simulink subsystem "Controllers"  (R2024b)
settings: Solver=VariableStepAuto  StartTime=0.0  StopTime=10.0  RelTol=1e-3
undefined symbols (not defined in the file): CarrierFreq, dend, DiscIntNeverNeededParam, freq_left, freq_right, Ll, nb_cell, numberOfCell, numd, P_AC, Rl, Tctrl, Ts, V_AC_sec
libraries: powerlib_extras x12, simulink x12
(part 2 of 4)

== system Controllers/pulsegen_VBC1/pulse_gen ==
  Vcell_ref : Inport
  pgmode : Inport  Port=2
  Carrier_generatorgood : Subsystem  Commented=on  mask{fs=freq_right, nr=12*0+10, nb_mod=numberOfCell, x=0, Ts=Ts}
      mask prompts: fs "PWM freqency"; nr "carrier frequence/PWM freq"; nb_mod "nb cell"; x "x_shift (0:nb_cell, better nb_cell/x_shift not integal)"; Ts "time"
      mask init:
      | fc=fs*nr;
      | fx=fc/(1+x/nb_mod/nr);
  Mux4 : Mux  Inputs=6
  PWM : Subsystem
  Unit Delay : UnitDelay  SampleTime=Ts  HasFrameUpgradeWarning=on
  carrier_gen : Subsystem  mask(carrier generation){fc=CarrierFreq, range=[ 1 -1], Ms=numberOfCell, Ns=numberOfCell}
      mask prompts: fc "carrier frequency (Hz)"; range "carrier signal range"; Ms "M signals"; Ns "Enter N if two consecutive signals shifted (1/N) cycle. Enter 1 if all signals are identical."
      mask help:
      | Generating M number of triangle carrier signal(s) at specific frequency.
      | Two consecutive signals are shifted (1/N) cycles.
      |
      | Example 1:
      | put carrier frequency = 1e3, M=1, it outputs 1 triangle carrier signal with frequency of 1k Hz.
      |
      | Example 2:
      | M=3, N=3, output 3 evenly interleaved carrier signals. ( 2nd signal lags  1st signal by 1/3 cycle ).
      |
      | Example 3:
      | M=3, N=-2.5, output 3 carrier signals. (2nd signal advances 1st signal by 1/2.5 cycle).
      |
      | Example 4:
      | M=3, N=1, output 3 identical carrier signals.
      mask init:
      | fc=max(eps,fc); %avoid devided by 0;
      | % Ns=max(eps,Ns); %avoid devided by 0;
      | if Ns==0    %if Ns==0, not interleaved
      |     Ns=1;
      | end;
      | Ms=max(1,floor(Ms))-1;
      | rep_seq_t=[0 0.5 1]/fc;
      | rep_seq_y=[range(1) range(2) range(1)];
      | 
      | 
      | X = [];
      | Y = [];
      | if (length(rep_seq_t) ~= length(rep_seq_y)),
      |   error('Length of time vector and output vector must be the same.')
      | end
      | dbl_rep_seq_t = double(rep_seq_t);
      | dbl_rep_seq_y = double(rep_seq_y);
      | period = max(dbl_rep_seq_t) - min(dbl_rep_seq_t);
      | period = slResolve(sprintf('%0.5g',period), gcbh);
      | [X, Y] = genRepeatingSequenceBlockIconData(dbl_rep_seq_t, dbl_rep_seq_y);
      | Noffset=-[0:Ms]/Ns*period;
      mask Help: web('https://wiki.opal-rt.com/display/MMCDOC/Carrier+Signal+Generation+Block')
      mask Display: plot(X, Y )
  A_pulse : Outport  VectorParamsAs1DForOutWhenUnconnected=off
  NLC : Outport  Port=2  VectorParamsAs1DForOutWhenUnconnected=off
  wires:
  Unit Delay/1 -> A_pulse/1
  carrier_gen/1(Out1) -> Mux4/1, Mux4/2, Mux4/3, Mux4/4, Mux4/5, Mux4/6
  Vcell_ref/1 -> PWM/2(Vcell_ref)
  PWM/1(Upper_gate) -> Unit Delay/1
  Mux4/1 -> PWM/1(carrier)
  pgmode/1 -> PWM/3(pgmode)
  PWM/2(NLCref) -> NLC/1

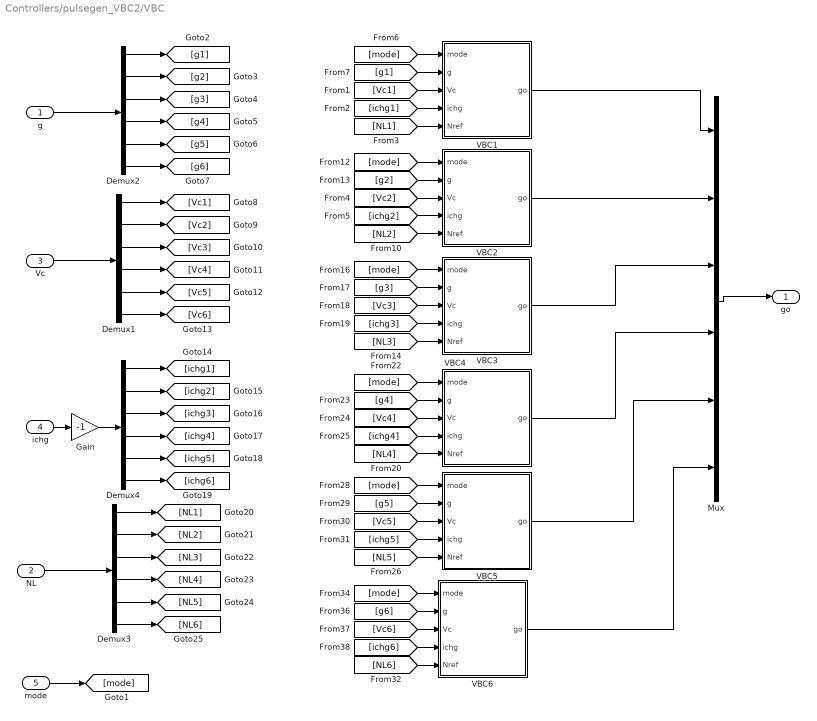
== system Controllers/pulsegen_VBC2/VBC ==
  g : Inport
  NL : Inport  Port=2
  Vc : Inport  Port=3
  ichg : Inport  Port=4
  mode : Inport  Port=5
  Demux{1..4} (4 alike) : Demux  Outputs=6
  Gain : Gain  Gain=-1
  Mux : Mux  Inputs=ones(6,1)*numberOfCell
  VBC1 : Subsystem
  VBC2 : Subsystem
  VBC3 : Subsystem
  VBC4 : Subsystem
  VBC5 : Subsystem
  VBC6 : Subsystem
  go : Outport  VectorParamsAs1DForOutWhenUnconnected=off
  wires:
  [NL6] -> VBC6/5(Nref)
  [ichg6] -> VBC6/4(ichg)
  [Vc6] -> VBC6/3(Vc)
  [g6] -> VBC6/2(g)
  [mode] -> VBC6/1(mode)
  [NL5] -> VBC5/5(Nref)
  [ichg5] -> VBC5/4(ichg)
  [Vc5] -> VBC5/3(Vc)
  [g5] -> VBC5/2(g)
  [mode] -> VBC5/1(mode)
  [NL4] -> VBC4/5(Nref)
  [ichg4] -> VBC4/4(ichg)
  [Vc4] -> VBC4/3(Vc)
  [g4] -> VBC4/2(g)
  [mode] -> VBC4/1(mode)
  [NL3] -> VBC3/5(Nref)
  [ichg3] -> VBC3/4(ichg)
  [Vc3] -> VBC3/3(Vc)
  [g3] -> VBC3/2(g)
  [mode] -> VBC3/1(mode)
  [NL2] -> VBC2/5(Nref)
  [ichg2] -> VBC2/4(ichg)
  [Vc2] -> VBC2/3(Vc)
  [g2] -> VBC2/2(g)
  [mode] -> VBC2/1(mode)
  [NL1] -> VBC1/5(Nref)
  [ichg1] -> VBC1/4(ichg)
  [Vc1] -> VBC1/3(Vc)
  Demux3/6 -> [NL6]
  Demux3/5 -> [NL5]
  Demux3/4 -> [NL4]
  Demux3/3 -> [NL3]
  Demux3/2 -> [NL2]
  Demux3/1 -> [NL1]
  NL/1 -> Demux3/1
  Demux4/6 -> [ichg6]
  Demux4/5 -> [ichg5]
  Demux4/4 -> [ichg4]
  Demux4/3 -> [ichg3]
  Demux4/2 -> [ichg2]
  Demux4/1 -> [ichg1]
  Demux1/6 -> [Vc6]
  Demux1/5 -> [Vc5]
  Demux1/4 -> [Vc4]
  Demux1/3 -> [Vc3]
  Demux1/2 -> [Vc2]
  Demux1/1 -> [Vc1]
  [g1] -> VBC1/2(g)
  Demux2/6 -> [g6]
  Demux2/5 -> [g5]
  Demux2/4 -> [g4]
  Demux2/3 -> [g3]
  Demux2/2 -> [g2]
  Demux2/1 -> [g1]
  [mode] -> VBC1/1(mode)
  mode/1 -> [mode]
  Gain/1 -> Demux4/1
  VBC1/1(go) -> Mux/1
  g/1 -> Demux2/1
  Vc/1 -> Demux1/1
  ichg/1 -> Gain/1
  VBC2/1(go) -> Mux/2
  VBC3/1(go) -> Mux/3
  VBC4/1(go) -> Mux/4
  VBC5/1(go) -> Mux/5
  VBC6/1(go) -> Mux/6
  Mux/1 -> go/1

== system Controllers/pulsegen_VBC2/pulse_gen ==
  Vcell_ref : Inport
  pgmode : Inport  Port=2
  Carrier_generatorgood : Subsystem  Commented=on  mask{fs=freq_right, nr=12*0+10, nb_mod=numberOfCell, x=0, Ts=Ts}
      mask prompts: fs "PWM freqency"; nr "carrier frequence/PWM freq"; nb_mod "nb cell"; x "x_shift (0:nb_cell, better nb_cell/x_shift not integal)"; Ts "time"
      mask init:
      | fc=fs*nr;
      | fx=fc/(1+x/nb_mod/nr);
  Memory2 : Memory  Commented=on
  Mux4 : Mux  Inputs=6
  PWM : Subsystem
  Unit Delay : UnitDelay  SampleTime=Ts  HasFrameUpgradeWarning=on
  carrier_gen : Subsystem  mask(carrier generation){fc=CarrierFreq, range=[ 1 -1], Ms=numberOfCell, Ns=numberOfCell}
      mask prompts: fc "carrier frequency (Hz)"; range "carrier signal range"; Ms "M signals"; Ns "Enter N if two consecutive signals shifted (1/N) cycle. Enter 1 if all signals are identical."
      mask help:
      | Generating M number of triangle carrier signal(s) at specific frequency.
      | Two consecutive signals are shifted (1/N) cycles.
      |
      | Example 1:
      | put carrier frequency = 1e3, M=1, it outputs 1 triangle carrier signal with frequency of 1k Hz.
      |
      | Example 2:
      | M=3, N=3, output 3 evenly interleaved carrier signals. ( 2nd signal lags  1st signal by 1/3 cycle ).
      |
      | Example 3:
      | M=3, N=-2.5, output 3 carrier signals. (2nd signal advances 1st signal by 1/2.5 cycle).
      |
      | Example 4:
      | M=3, N=1, output 3 identical carrier signals.
      mask init: same as Controllers/pulsegen_VBC1/pulse_gen/carrier_gen
      mask Help: web('https://wiki.opal-rt.com/display/MMCDOC/Carrier+Signal+Generation+Block')
      mask Display: plot(X, Y )
  A_pulse : Outport  VectorParamsAs1DForOutWhenUnconnected=off
  NLC : Outport  Port=2  VectorParamsAs1DForOutWhenUnconnected=off
  wires:
  Unit Delay/1 -> A_pulse/1
  carrier_gen/1(Out1) -> Mux4/6, Mux4/5, Mux4/4, Mux4/3, Mux4/2, Mux4/1
  PWM/2(NLCref) -> NLC/1
  pgmode/1 -> PWM/3(pgmode)
  Mux4/1 -> PWM/1(carrier)
  Carrier_generatorgood/1(Out1) -> ?
  PWM/1(Upper_gate) -> Unit Delay/1
  Vcell_ref/1 -> PWM/2(Vcell_ref)

== system Controllers/sorting Tmuxed/demux ==
  enable : Inport
  data : Inport  Port=2
  Mux : Mux  Inputs=ones(6,1)*numberOfCell
  Subsystem1 : Subsystem
  Subsystem2 : Subsystem
  Subsystem3 : Subsystem
  Subsystem4 : Subsystem
  Subsystem5 : Subsystem
  Subsystem6 : Subsystem
  Unit Delay{,1..5} (6 alike) : UnitDelay  SampleTime=Ts  HasFrameUpgradeWarning=on
  do : Outport  VectorParamsAs1DForOutWhenUnconnected=off
  endly : Outport  Port=2  VectorParamsAs1DForOutWhenUnconnected=off
  wires:
  Unit Delay5/1 -> endly/1
  data/1 -> Subsystem5/1(In1), Subsystem6/1(In1), Subsystem3/1(In1), Subsystem2/1(In1), Subsystem1/1(In1), Subsystem4/1(In1)
  Subsystem4/1(Out1) -> Mux/1
  Subsystem1/1(Out1) -> Mux/2
  Subsystem2/1(Out1) -> Mux/3
  Subsystem3/1(Out1) -> Mux/4
  Subsystem5/1(Out1) -> Mux/5
  Subsystem6/1(Out1) -> Mux/6
  Mux/1 -> do/1
  enable/1 -> Subsystem4/Enable, Unit Delay/1
  Unit Delay/1 -> Subsystem1/Enable, Unit Delay1/1
  Unit Delay1/1 -> Unit Delay2/1, Subsystem2/Enable
  Unit Delay2/1 -> Subsystem3/Enable, Unit Delay3/1
  Unit Delay3/1 -> Subsystem5/Enable, Unit Delay4/1
  Unit Delay4/1 -> Subsystem6/Enable, Unit Delay5/1

== system Controllers/sorting Tmuxed/demux1 ==
  enable : Inport
  data : Inport  Port=2
  Mux : Mux  Inputs=ones(6,1)*numberOfCell
  Subsystem1 : Subsystem
  Subsystem2 : Subsystem
  Subsystem3 : Subsystem
  Subsystem4 : Subsystem
  Subsystem5 : Subsystem
  Subsystem6 : Subsystem
  Unit Delay{,1..5} (6 alike) : UnitDelay  SampleTime=Ts  HasFrameUpgradeWarning=on
  do : Outport  VectorParamsAs1DForOutWhenUnconnected=off
  endly : Outport  Port=2  VectorParamsAs1DForOutWhenUnconnected=off
  wires:
  Unit Delay4/1 -> Unit Delay5/1, Subsystem6/Enable
  Unit Delay3/1 -> Unit Delay4/1, Subsystem5/Enable
  Unit Delay2/1 -> Unit Delay3/1, Subsystem3/Enable
  Unit Delay1/1 -> Subsystem2/Enable, Unit Delay2/1
  Unit Delay/1 -> Unit Delay1/1, Subsystem1/Enable
  enable/1 -> Unit Delay/1, Subsystem4/Enable
  Mux/1 -> do/1
  Subsystem6/1(Out1) -> Mux/6
  Subsystem5/1(Out1) -> Mux/5
  Subsystem3/1(Out1) -> Mux/4
  Subsystem2/1(Out1) -> Mux/3
  Subsystem1/1(Out1) -> Mux/2
  Subsystem4/1(Out1) -> Mux/1
  data/1 -> Subsystem4/1(In1), Subsystem1/1(In1), Subsystem2/1(In1), Subsystem3/1(In1), Subsystem6/1(In1), Subsystem5/1(In1)
  Unit Delay5/1 -> endly/1

== system Controllers/Subsystem/Subsystem1/Subsystem1 ==
  In1 : Inport
  inx : Inport  Port=2
  Selector : Selector  InputPortWidth=200  IndexOptions=Index vector (port)  Indices=[1 3]  OutputSizes=1
  Out1 : Outport  VectorParamsAs1DForOutWhenUnconnected=off
  wires:
  In1/1 -> Selector/1
  Selector/1 -> Out1/1
  inx/1 -> Selector/2

== system Controllers/Subsystem/Subsystem1/Subsystem2 ==
  In1 : Inport
  inx : Inport  Port=2
  Selector : Selector  InputPortWidth=200  IndexOptions=Index vector (port)  Indices=[1 3]  OutputSizes=1
  Out1 : Outport  VectorParamsAs1DForOutWhenUnconnected=off
  wires:
  inx/1 -> Selector/2
  Selector/1 -> Out1/1
  In1/1 -> Selector/1

== system Controllers/Subsystem/Subsystem1/Subsystem3 ==
  In1 : Inport
  inx : Inport  Port=2
  Selector : Selector  InputPortWidth=200  IndexOptions=Index vector (port)  Indices=[1 3]  OutputSizes=1
  Out1 : Outport  VectorParamsAs1DForOutWhenUnconnected=off
  wires:
  inx/1 -> Selector/2
  Selector/1 -> Out1/1
  In1/1 -> Selector/1

== system Controllers/Subsystem/Subsystem1/Subsystem4 ==
  In1 : Inport
  inx : Inport  Port=2
  Selector : Selector  InputPortWidth=200  IndexOptions=Index vector (port)  Indices=[1 3]  OutputSizes=1
  Out1 : Outport  VectorParamsAs1DForOutWhenUnconnected=off
  wires:
  In1/1 -> Selector/1
  Selector/1 -> Out1/1
  inx/1 -> Selector/2

== system Controllers/Subsystem/Subsystem1/Subsystem5 ==
  In1 : Inport
  inx : Inport  Port=2
  Selector : Selector  InputPortWidth=200  IndexOptions=Index vector (port)  Indices=[1 3]  OutputSizes=1
  Out1 : Outport  VectorParamsAs1DForOutWhenUnconnected=off
  wires:
  inx/1 -> Selector/2
  Selector/1 -> Out1/1
  In1/1 -> Selector/1

== system Controllers/Subsystem/Subsystem1/Subsystem6 ==
  In1 : Inport
  inx : Inport  Port=2
  Selector : Selector  InputPortWidth=200  IndexOptions=Index vector (port)  Indices=[1 3]  OutputSizes=1
  Out1 : Outport  VectorParamsAs1DForOutWhenUnconnected=off
  wires:
  In1/1 -> Selector/1
  Selector/1 -> Out1/1
  inx/1 -> Selector/2

== system Controllers/Subsystem/Subsystem3/Subsystem1 ==
  In1 : Inport
  MinMax : MinMax
  MinMax1 : MinMax  Function=max
  Mux : Mux  Inputs=3
  Sum of Elements : Sum  Inputs=+
  Vc_SI_to_pu1 : Gain  Gain=1/(nb_cell/2)  SampleTime=Tctrl
  Out1 : Outport  VectorParamsAs1DForOutWhenUnconnected=off
  wires:
  Sum of Elements/1 -> Vc_SI_to_pu1/1
  MinMax1/1 -> Mux/2
  Mux/1 -> Out1/1
  MinMax/1 -> Mux/1
  In1/1 -> MinMax1/1, MinMax/1, Sum of Elements/1
  Vc_SI_to_pu1/1 -> Mux/3

== system Controllers/Subsystem/Subsystem3/Subsystem2 ==
  In1 : Inport
  MinMax : MinMax
  MinMax1 : MinMax  Function=max
  Mux : Mux  Inputs=3
  Sum of Elements : Sum  Inputs=+
  Vc_SI_to_pu1 : Gain  Gain=1/(nb_cell/2)  SampleTime=Tctrl
  Out1 : Outport  VectorParamsAs1DForOutWhenUnconnected=off
  wires:
  Vc_SI_to_pu1/1 -> Mux/3
  In1/1 -> Sum of Elements/1, MinMax/1, MinMax1/1
  MinMax/1 -> Mux/1
  Mux/1 -> Out1/1
  MinMax1/1 -> Mux/2
  Sum of Elements/1 -> Vc_SI_to_pu1/1

== system Controllers/Subsystem/Subsystem3/Subsystem3 ==
  In1 : Inport
  MinMax : MinMax
  MinMax1 : MinMax  Function=max
  Mux : Mux  Inputs=3
  Sum of Elements : Sum  Inputs=+
  Vc_SI_to_pu1 : Gain  Gain=1/(nb_cell/2)  SampleTime=Tctrl
  Out1 : Outport  VectorParamsAs1DForOutWhenUnconnected=off
  wires:
  Vc_SI_to_pu1/1 -> Mux/3
  In1/1 -> Sum of Elements/1, MinMax/1, MinMax1/1
  MinMax/1 -> Mux/1
  Mux/1 -> Out1/1
  MinMax1/1 -> Mux/2
  Sum of Elements/1 -> Vc_SI_to_pu1/1

== system Controllers/Subsystem/Subsystem3/Subsystem4 ==
  In1 : Inport
  MinMax : MinMax
  MinMax1 : MinMax  Function=max
  Mux : Mux  Inputs=3
  Sum of Elements : Sum  Inputs=+
  Vc_SI_to_pu1 : Gain  Gain=1/(nb_cell/2)  SampleTime=Tctrl
  Out1 : Outport  VectorParamsAs1DForOutWhenUnconnected=off
  wires:
  Vc_SI_to_pu1/1 -> Mux/3
  In1/1 -> Sum of Elements/1, MinMax/1, MinMax1/1
  MinMax/1 -> Mux/1
  Mux/1 -> Out1/1
  MinMax1/1 -> Mux/2
  Sum of Elements/1 -> Vc_SI_to_pu1/1

== system Controllers/Subsystem/Subsystem3/Subsystem5 ==
  In1 : Inport
  MinMax : MinMax
  MinMax1 : MinMax  Function=max
  Mux : Mux  Inputs=3
  Sum of Elements : Sum  Inputs=+
  Vc_SI_to_pu1 : Gain  Gain=1/(nb_cell/2)  SampleTime=Tctrl
  Out1 : Outport  VectorParamsAs1DForOutWhenUnconnected=off
  wires:
  Sum of Elements/1 -> Vc_SI_to_pu1/1
  MinMax1/1 -> Mux/2
  Mux/1 -> Out1/1
  MinMax/1 -> Mux/1
  In1/1 -> MinMax1/1, MinMax/1, Sum of Elements/1
  Vc_SI_to_pu1/1 -> Mux/3

== system Controllers/Subsystem/Subsystem3/Subsystem6 ==
  In1 : Inport
  MinMax : MinMax
  MinMax1 : MinMax  Function=max
  Mux : Mux  Inputs=3
  Sum of Elements : Sum  Inputs=+
  Vc_SI_to_pu1 : Gain  Gain=1/(nb_cell/2)  SampleTime=Tctrl
  Out1 : Outport  VectorParamsAs1DForOutWhenUnconnected=off
  wires:
  Sum of Elements/1 -> Vc_SI_to_pu1/1
  MinMax1/1 -> Mux/2
  Mux/1 -> Out1/1
  MinMax/1 -> Mux/1
  In1/1 -> MinMax1/1, MinMax/1, Sum of Elements/1
  Vc_SI_to_pu1/1 -> Mux/3

== system Controllers/Subsystem2/Subsystem/Subsystem3 ==
  vi_ac : Inport
  3-phase Instantaneous Active & Reactive Power : powerlib_extras/Measurements/3-phase  Instantaneous  Active & Reactive Power
  Demux3 : Demux  Outputs=[3 3 ]
  Gain1 : Gain  Gain=1/V_AC_sec*sqrt(3/2)
  Gain2 : Gain  Gain=2/3
  Gain4 : Gain  Gain=V_AC_sec/P_AC*sqrt(3/2)
  "vabc_pu " : Outport  VectorParamsAs1DForOutWhenUnconnected=off
  Iabc_pu : Outport  Port=2  VectorParamsAs1DForOutWhenUnconnected=off
  PQpu : Outport  Port=3  VectorParamsAs1DForOutWhenUnconnected=off
  wires:
  Gain2/1 -> PQpu/1
  Demux3/1 -> Gain1/1
  vi_ac/1 -> Demux3/1
  Demux3/2 -> Gain4/1
  3-phase Instantaneous Active & Reactive Power/1 -> Gain2/1
  Gain1/1 -> 3-phase Instantaneous Active & Reactive Power/1, "vabc_pu "/1
  Gain4/1 -> 3-phase Instantaneous Active & Reactive Power/2, Iabc_pu/1

== system Controllers/Subsystem2/Subsystem/Subsystem4 ==
  vi_ac : Inport
  3-phase Instantaneous Active & Reactive Power : powerlib_extras/Measurements/3-phase  Instantaneous  Active & Reactive Power
  Demux3 : Demux  Outputs=[3 3 ]
  Gain1 : Gain  Gain=1/V_AC_sec*sqrt(3/2)
  Gain2 : Gain  Gain=2/3
  Gain4 : Gain  Gain=V_AC_sec/P_AC*sqrt(3/2)
  "vabc_pu " : Outport  VectorParamsAs1DForOutWhenUnconnected=off
  Iabc_pu : Outport  Port=2  VectorParamsAs1DForOutWhenUnconnected=off
  PQpu : Outport  Port=3  VectorParamsAs1DForOutWhenUnconnected=off
  wires:
  Gain4/1 -> Iabc_pu/1, 3-phase Instantaneous Active & Reactive Power/2
  Gain1/1 -> "vabc_pu "/1, 3-phase Instantaneous Active & Reactive Power/1
  3-phase Instantaneous Active & Reactive Power/1 -> Gain2/1
  Demux3/2 -> Gain4/1
  vi_ac/1 -> Demux3/1
  Demux3/1 -> Gain1/1
  Gain2/1 -> PQpu/1

== system Controllers/VSC controller1/Vdc ctrl/Vdc_ctrler1 ==
  Vcap : Inport
  Enable : EnablePort  StatesWhenEnabling=reset
  Add2 : Sum  Inputs=+-
  PI_d2 : Subsystem  AncestorBlock=|  DialogController=POWERSYS.PowerSysDialog  mask(Discrete PI Controller){Kp=Kvdc(1), Ki=Kvdc(2), Par_Limits=[1 -1]*0.3, Init=0, Ts=Ts}
      | powerlib_extras/Discrete 
      | Control Blocks/Discrete
      | PI Controller
      mask prompts: Kp "Proportional gain (Kp):"; Ki "Integral gain (Ki):"; Par_Limits "Output limits: [ Upper   Lower ]"; Init "Output initial value:"; Ts "Sample time:"
      mask help: This block implements a discrete PI controller.
      mask init:
      | UpperLimit=Par_Limits(1);
      | LowerLimit=Par_Limits(2);
      | power_initmask();
      mask Help: This block is part of a subset of blocks in the Extras library that does not have documentation associated with it, other than the block mask description.
      mask Display: disp('PI');
  Saturation : Saturate  UpperLimit=0.1  LowerLimit=-0.1
      settings: AttributesFormatString=%<LowerLimit>~%<UpperLimit>
  Vdcpuref : Constant
  Vdctrl : Scope  NumInputPorts=2
  delP : Outport  OutputWhenDisabled=reset  InitialOutput=[0]  VectorParamsAs1DForOutWhenUnconnected=off
  wires:
  Add2/1 -> Saturation/1  "delVdc"
  Vcap/1 -> Vdctrl/1, Add2/1
  Vdcpuref/1 -> Add2/2
  Saturation/1 -> PI_d2/1(Error)
  PI_d2/1(Out) -> Vdctrl/2, delP/1  "PIVdc"

== system Controllers/VSC controller1/Vdc ctrl/moded ==
  Vcap : Inport
  Vdc : Inport  Port=2
  Compare To Constant : simulink/Logic and Bit Operations/Compare To Constant  relop=>=  const=1.05  OutDataTypeStr=uint8
  Compare To Constant1 : simulink/Logic and Bit Operations/Compare To Constant  relop=<=  const=0.95  OutDataTypeStr=uint8
  Logical Operator1 : Logic  Operator=OR  Inputs=1  AllPortsSameDT=off  OutDataTypeStr=boolean
  Mux1 : Mux  Inputs=2
  Mux9 : Mux  Inputs=2
  Nmode : Outport  VectorParamsAs1DForOutWhenUnconnected=off
  wires:
  Mux9/1 -> Compare To Constant1/1, Compare To Constant/1
  Compare To Constant/1 -> Mux1/1
  Compare To Constant1/1 -> Mux1/2
  Mux1/1 -> Logical Operator1/1
  Vcap/1 -> Mux9/1
  Vdc/1 -> Mux9/2
  Logical Operator1/1 -> Nmode/1

== system Controllers/VSC controller1/otherctrl/3to6 ==
  In1 : Inport
  Gain2 : Gain  Gain=-1
  Mux : Mux  Inputs=2
  phase_reorder2 : Selector  InputPortWidth=6  IndexOptions=Index vector (dialog)  Indices=[1 4 2 5 3 6 ]  OutputSizes=1
  Out1 : Outport  VectorParamsAs1DForOutWhenUnconnected=off
  wires:
  Mux/1 -> phase_reorder2/1  "a1b1c1a2b2c2"
  In1/1 -> Mux/2, Gain2/1
  Gain2/1 -> Mux/1
  phase_reorder2/1 -> Out1/1  "a1a2b1b2c1c2"

== system Controllers/VSC controller1/otherctrl/VSCController_ctrl ==
  Vac_ref : Inport
  hisi_VcLP : Inport  Port=2
  Vcap : Inport  Port=3
  mode : Inport  Port=4
  Iarm : Inport  Port=5
  Idc0 : Inport  Port=6
  P_ref : Inport  Port=7
  vdcref : Inport  Port=8
  theda_eVLP : Inport  Port=9
  Lx_ctrl3 : Inport  Port=10
  ctrlI : Inport  Port=11
  ver : Inport  Port=12
  Ts : Inport  Port=13
  Bus Creator : BusCreator  Inputs=12
  Bus Selector1 : BusSelector  OutputSignals=Vac_ref,VcapLP2;hisi,Vcap,mode,Iarm,vdcref,enblVcLP;theda,xtrIctrl3,Ictrl,Ts
  ver2 : Subsystem
  ref : Outport
  hiso : Outport  Port=2  InitialOutput=0
  wires:
  Bus Selector1/8 -> ver2/8(Lxpu)  "<xtrIctrl3>"
  ver2/1(ref) -> ref/1
  Bus Selector1/10 -> ver2/10(Ts)  "<Ts>"
  Bus Selector1/9 -> ver2/9(Ictrl)  "<Ictrl>"
  Bus Selector1/7 -> ver2/7(theda)  "<enblVcLP;theda>"
  Bus Selector1/6 -> ver2/6(vdcref)  "<vdcref>"
  Bus Selector1/5 -> ver2/5(Iarm)  "<Iarm>"
  Bus Selector1/4 -> ver2/4(mode)  "<mode>"
  Bus Selector1/3 -> ver2/3(Vcap)  "<Vcap>"
  Bus Selector1/2 -> ver2/2(hisi)  "<VcapLP2;hisi>"
  Bus Selector1/1 -> ver2/1(Vac_ref)  "<Vac_ref>"
  Bus Creator/1 -> Bus Selector1/1
  Ts/1 -> Bus Creator/12  "Ts"
  Lx_ctrl3/1 -> Bus Creator/10  "xtrIctrl3"
  vdcref/1 -> Bus Creator/8  "vdcref"
  Idc0/1 -> Bus Creator/6  "Idc0"
  mode/1 -> Bus Creator/4  "mode"
  hisi_VcLP/1 -> Bus Creator/2  "VcapLP2;hisi"
  Vac_ref/1 -> Bus Creator/1  "Vac_ref"
  Vcap/1 -> Bus Creator/3  "Vcap"
  Iarm/1 -> Bus Creator/5  "Iarm"
  P_ref/1 -> Bus Creator/7  "P_ref"
  theda_eVLP/1 -> Bus Creator/9  "enblVcLP;theda"
  ctrlI/1 -> Bus Creator/11  "Ictrl"
  ver2/2(hiso) -> hiso/1

== system Controllers/VSC controller1/otherctrl/cur-cal ==
  In1 : Inport
  Demux3 : Demux  Outputs=6
  Gain14 : Gain  Gain=0.5
  Mux3 : Mux  Inputs=3
  Sum10 : Sum  Inputs=2
  Sum11 : Sum  Inputs=2
  Sum9 : Sum  Inputs=2
  V--> pu_AC_sec1 : Gain  Gain=1/(Sb/(Vb*sqrt(3))*sqrt(2)/2+Sb/(Vdc*2)/3)
  Out1 : Outport  VectorParamsAs1DForOutWhenUnconnected=off
  wires:
  Gain14/1 -> Out1/1
  In1/1 -> V--> pu_AC_sec1/1
  V--> pu_AC_sec1/1 -> Demux3/1
  Mux3/1 -> Gain14/1
  Sum10/1 -> Mux3/3
  Sum9/1 -> Mux3/1
  Demux3/6 -> Sum11/2
  Sum11/1 -> Mux3/2
  Demux3/5 -> Sum11/1
  Demux3/4 -> Sum10/2
  Demux3/3 -> Sum10/1
  Demux3/2 -> Sum9/2
  Demux3/1 -> Sum9/1

== system Controllers/VSC controller1/pqctrl/Ramp2 ==
  y* : Inport
  J/Psi : Gain  SaturateOnIntegerOverflow=on  OutDataTypeStr=Inherit: Same as input  ParamDataTypeStr=Inherit: Same as input
  Saturation : Saturate  UpperLimit=ramp*Ts  LowerLimit=-ramp*Ts
  Sum : Sum  Inputs=|++  InputSameDT=on  SaturateOnIntegerOverflow=on  OutDataTypeStr=Inherit: Same as first input
  Sum1 : Sum  Inputs=|+-  InputSameDT=on  SaturateOnIntegerOverflow=on  OutDataTypeStr=Inherit: Same as first input
  Unit Delay : UnitDelay  SampleTime=Ts  HasFrameUpgradeWarning=on
  yramp* : Outport  VectorParamsAs1DForOutWhenUnconnected=off
  wires:
  Unit Delay/1 -> Sum1/2, Sum/2
  J/Psi/1 -> Unit Delay/1
  Sum1/1 -> Saturation/1
  Saturation/1 -> Sum/1
  Sum/1 -> yramp*/1, J/Psi/1
  y*/1 -> Sum1/1

== system Controllers/VSC controller1/pqctrl/dq ctlr ==
  Vabcpu : Inport
  iabcpu : Inport  Port=2
  theda : Inport  Port=3
  PQrefpu : Inport  Port=4
  Demux : Demux  Outputs=2
  Gain1 : Gain  Gain=1/ks
  Mux3 : Mux  Inputs=2
  PI_d1 : powerlib_extras/Discrete  Control Blocks/Discrete PI Controller  Kp=Kp(1)  Ki=Kp(2)  Par_Limits=[1 -1]*0.15  Init=0  Ts=Ts
  PI_d2 : powerlib_extras/Discrete  Control Blocks/Discrete PI Controller  Kp=Kd(1)  Ki=Kd(2)  Par_Limits=[1 -1]*0.25  Init=0  Ts=Ts
  Subsystem1 : Subsystem
  Subtract : Sum  Inputs=+-
  Subtract1 : Sum
  Subtract2 : Sum  Commented=on  Inputs=+-
  Vdqref : Subsystem
  abc_dq : Subsystem
  abc_dq1 : Subsystem
  measure : Subsystem  Commented=on
  Vdqpu : Outport  VectorParamsAs1DForOutWhenUnconnected=off
  wires:
  Gain1/1 -> Vdqpu/1  "Vdqpu"
  iabcpu/1 -> abc_dq1/1(abc)  "iabc"
  PQrefpu/1 -> Subsystem1/2(PQref)
  theda/1 -> abc_dq1/2(theta), abc_dq/2(theta)
  Vabcpu/1 -> abc_dq/1(abc)  "vabc"
  Subtract1/1 -> Gain1/1, Subtract2/1
  Mux3/1 -> Subtract1/2
  PI_d1/1 -> Mux3/2
  PI_d2/1 -> Mux3/1
  Vdqref/1(Vdqrefss) -> Subtract1/1
  Demux/2 -> PI_d1/1
  Demux/1 -> PI_d2/1
  Subtract/1 -> Demux/1
  abc_dq1/1(dq) -> Subtract/2  "idq"
  abc_dq/1(dq) -> Subsystem1/1(Vdq2), Vdqref/1(Vdq2), Subtract2/2  "Vdq"
  Subsystem1/1(Idqref) -> Subtract/1, Vdqref/2(Idqref), measure/2(Idqref)  "idqref"
  Subtract2/1 -> measure/1(A=X-V)

== system Controllers/VSC controller1/pqctrl/dq->abc ==
  note: Vc= Vd*sin(wt+2pi/3) + Vq*cos(wt+2pi/3) + Vo
  note: Vb= Vd*sin(wt-2pi/3) + Vq*cos(wt-2pi/3) + Vo
  note: Va= Vd*sinwt + Vq*cos(wt) + Vo
  dq : Inport
  theda : Inport  Port=2
  Fcn : Fcn  Expr=(u(1)*sin(u(3))+u(2)*cos(u(3)))
  Fcn1 : Fcn  Expr=(u(1)*sin(u(3)-2*pi/3)+u(2)*cos(u(3)-2*pi/3))
  Fcn2 : Fcn  Expr=(u(1)*sin(u(3)+2*pi/3)+u(2)*cos(u(3)+2*pi/3))
  Mux1 : Mux  Inputs=2
  Mux3 : Mux  Inputs=3
  abc : Outport  VectorParamsAs1DForOutWhenUnconnected=off
  wires:
  Mux3/1 -> abc/1  "abc"
  theda/1 -> Mux1/2
  dq/1 -> Mux1/1
  Mux1/1 -> Fcn1/1, Fcn2/1, Fcn/1
  Fcn/1 -> Mux3/1
  Fcn1/1 -> Mux3/2
  Fcn2/1 -> Mux3/3

== system Controllers/VSC controller1/pqctrl/satuation on amplitute  ==
  Vdq : Inport
  limitVdq : Inport  Port=2
  "Bias important; cancel delay in control cycle, so the PI(error) is zero, other wise PI(errer) is bais, which could over limit" : Bias  Bias=nadv*Ts*2*pi*frq  SaturateOnIntegerOverflow=off
  Complex to Magnitude-Angle : ComplexToMagnitudeAngle
  Complex to Real-Imag : ComplexToRealImag
  Demux1 : Demux  Outputs=2
  Gain : Gain  Gain=-1
  Magnitude-Angle to Complex : MagnitudeAngleToComplex
  Mux4 : Mux  Inputs=2
  Real-Imag to Complex : RealImagToComplex
  Saturation Dynamic : simulink/Discontinuities/Saturation Dynamic  OutMin=[]  OutMax=[]  OutDataTypeStr=Inherit: Same as second input  OutDataType=fixdt(1, 16)  OutScaling=2^-10  DoSatur=off
  Out1 : Outport  VectorParamsAs1DForOutWhenUnconnected=off
  wires:
  Vdq/1 -> Demux1/1
  Mux4/1 -> Out1/1
  Complex to Real-Imag/1 -> Mux4/1
  Complex to Real-Imag/2 -> Mux4/2
  Magnitude-Angle to Complex/1 -> Complex to Real-Imag/1
  Complex to Magnitude-Angle/2 -> "Bias important; cancel delay in control cycle, so the PI(error) is zero, other wise PI(errer) is bais, which could over limit"/1
  Real-Imag to Complex/1 -> Complex to Magnitude-Angle/1
  Demux1/2 -> Real-Imag to Complex/2
  Demux1/1 -> Real-Imag to Complex/1
  Saturation Dynamic/1 -> Magnitude-Angle to Complex/1
  Complex to Magnitude-Angle/1 -> Saturation Dynamic/2
  limitVdq/1 -> Saturation Dynamic/1, Gain/1
  Gain/1 -> Saturation Dynamic/3
  "Bias important; cancel delay in control cycle, so the PI(error) is zero, other wise PI(errer) is bais, which could over limit"/1 -> Magnitude-Angle to Complex/2

== system Controllers/VSC controller1/pqctrl/vipqscope ==
  note: Iacpu
  note: Iacpu
  Vac : Inport
  Iac : Inport  Port=2
  pqref : Inport  Port=3
  3-phase Instantaneous Active & Reactive Power : powerlib_extras/Measurements/3-phase  Instantaneous  Active & Reactive Power
  Demux1 : Demux  Outputs=2
  Demux2 : Demux  Outputs=2
  Gain2 : Gain  Gain=2/3
  Mux1 : Mux  Inputs=2
  Mux3 : Mux  Inputs=2
  vipq : Scope  Commented=on  NumInputPorts=4
  wires:
  pqref/1 -> Demux1/1
  Demux1/2 -> Mux3/1
  Iac/1 -> 3-phase Instantaneous Active & Reactive Power/2, vipq/2
  Vac/1 -> 3-phase Instantaneous Active & Reactive Power/1, vipq/1  "Vacpu"
  Demux1/1 -> Mux1/1
  3-phase Instantaneous Active & Reactive Power/1 -> Gain2/1
  Gain2/1 -> Demux2/1
  Demux2/1 -> Mux1/2
  Demux2/2 -> Mux3/2
  Mux3/1 -> vipq/4  "q"
  Mux1/1 -> vipq/3  "p"

== system Controllers/VSC controller2/Vdc ctrl/Vdc_ctrler1 ==
  Vcap : Inport
  Enable : EnablePort  StatesWhenEnabling=reset
  Add2 : Sum  Inputs=+-
  PI_d2 : Subsystem  AncestorBlock=|  DialogController=POWERSYS.PowerSysDialog  mask(Discrete PI Controller){Kp=Kvdc(1), Ki=Kvdc(2), Par_Limits=[1 -1]*0.3, Init=0, Ts=Ts}
      | powerlib_extras/Discrete 
      | Control Blocks/Discrete
      | PI Controller
      mask prompts: Kp "Proportional gain (Kp):"; Ki "Integral gain (Ki):"; Par_Limits "Output limits: [ Upper   Lower ]"; Init "Output initial value:"; Ts "Sample time:"
      mask help: This block implements a discrete PI controller.
      mask init:
      | UpperLimit=Par_Limits(1);
      | LowerLimit=Par_Limits(2);
      | power_initmask();
      mask Help: This block is part of a subset of blocks in the Extras library that does not have documentation associated with it, other than the block mask description.
      mask Display: disp('PI');
  Saturation : Saturate  UpperLimit=0.1  LowerLimit=-0.1
      settings: AttributesFormatString=%<LowerLimit>~%<UpperLimit>
  Vdcpuref : Constant
  Vdctrl : Scope  NumInputPorts=2
  delP : Outport  OutputWhenDisabled=reset  InitialOutput=[0]  VectorParamsAs1DForOutWhenUnconnected=off
  wires:
  PI_d2/1(Out) -> delP/1, Vdctrl/2  "PIVdc"
  Saturation/1 -> PI_d2/1(Error)
  Vdcpuref/1 -> Add2/2
  Vcap/1 -> Add2/1, Vdctrl/1
  Add2/1 -> Saturation/1  "delVdc"

== system Controllers/VSC controller2/Vdc ctrl/moded ==
  Vcap : Inport
  Vdc : Inport  Port=2
  Compare To Constant : simulink/Logic and Bit Operations/Compare To Constant  relop=>=  const=1.05  OutDataTypeStr=uint8
  Compare To Constant1 : simulink/Logic and Bit Operations/Compare To Constant  relop=<=  const=0.95  OutDataTypeStr=uint8
  Logical Operator1 : Logic  Operator=OR  Inputs=1  AllPortsSameDT=off  OutDataTypeStr=boolean
  Mux1 : Mux  Inputs=2
  Mux9 : Mux  Inputs=2
  Nmode : Outport  VectorParamsAs1DForOutWhenUnconnected=off
  wires:
  Logical Operator1/1 -> Nmode/1
  Vdc/1 -> Mux9/2
  Vcap/1 -> Mux9/1
  Mux1/1 -> Logical Operator1/1
  Compare To Constant1/1 -> Mux1/2
  Compare To Constant/1 -> Mux1/1
  Mux9/1 -> Compare To Constant/1, Compare To Constant1/1

== system Controllers/VSC controller2/otherctrl/3to6 ==
  In1 : Inport
  Gain2 : Gain  Gain=-1
  Mux : Mux  Inputs=2
  phase_reorder2 : Selector  InputPortWidth=6  IndexOptions=Index vector (dialog)  Indices=[1 4 2 5 3 6 ]  OutputSizes=1
  Out1 : Outport  VectorParamsAs1DForOutWhenUnconnected=off
  wires:
  phase_reorder2/1 -> Out1/1  "a1a2b1b2c1c2"
  Gain2/1 -> Mux/1
  In1/1 -> Gain2/1, Mux/2
  Mux/1 -> phase_reorder2/1  "a1b1c1a2b2c2"

== system Controllers/VSC controller2/otherctrl/VSCController_ctrl ==
  Vac_ref : Inport
  hisi_VcLP : Inport  Port=2
  Vcap : Inport  Port=3
  mode : Inport  Port=4
  Iarm : Inport  Port=5
  Idc0 : Inport  Port=6
  P_ref : Inport  Port=7
  vdcref : Inport  Port=8
  theda_eVLP : Inport  Port=9
  Lx_ctrl3 : Inport  Port=10
  ctrlI : Inport  Port=11
  Ts : Inport  Port=12
  Bus Creator : BusCreator  Inputs=12
  Bus Selector1 : BusSelector  OutputSignals=Vac_ref,VcapLP2;hisi,Vcap,mode,Iarm,vdcref,enblVcLP;theda,xtrIctrl3,Ictrl,Ts
  ver2 : Subsystem
  ref : Outport
  hiso : Outport  Port=2  InitialOutput=0
  wires:
  ver2/1(ref) -> ref/1
  Bus Selector1/8 -> ver2/8(Lxpu)  "<xtrIctrl3>"
  Bus Selector1/10 -> ver2/10(Ts)  "<Ts>"
  Bus Selector1/9 -> ver2/9(Ictrl)  "<Ictrl>"
  Bus Selector1/7 -> ver2/7(theda)  "<enblVcLP;theda>"
  Bus Selector1/6 -> ver2/6(vdcref)  "<vdcref>"
  Bus Selector1/5 -> ver2/5(Iarm)  "<Iarm>"
  Bus Selector1/4 -> ver2/4(mode)  "<mode>"
  Bus Selector1/3 -> ver2/3(Vcap)  "<Vcap>"
  Bus Selector1/2 -> ver2/2(hisi)  "<VcapLP2;hisi>"
  Bus Selector1/1 -> ver2/1(Vac_ref)  "<Vac_ref>"
  Bus Creator/1 -> Bus Selector1/1
  Ts/1 -> Bus Creator/12  "Ts"
  Lx_ctrl3/1 -> Bus Creator/10  "xtrIctrl3"
  vdcref/1 -> Bus Creator/8  "vdcref"
  Idc0/1 -> Bus Creator/6  "Idc0"
  mode/1 -> Bus Creator/4  "mode"
  hisi_VcLP/1 -> Bus Creator/2  "VcapLP2;hisi"
  Vac_ref/1 -> Bus Creator/1  "Vac_ref"
  Vcap/1 -> Bus Creator/3  "Vcap"
  Iarm/1 -> Bus Creator/5  "Iarm"
  P_ref/1 -> Bus Creator/7  "P_ref"
  theda_eVLP/1 -> Bus Creator/9  "enblVcLP;theda"
  ctrlI/1 -> Bus Creator/11  "Ictrl"
  ver2/2(hiso) -> hiso/1

== system Controllers/VSC controller2/otherctrl/cur-cal ==
  In1 : Inport
  Demux3 : Demux  Outputs=6
  Gain14 : Gain  Gain=0.5
  Mux3 : Mux  Inputs=3
  Sum10 : Sum  Inputs=2
  Sum11 : Sum  Inputs=2
  Sum9 : Sum  Inputs=2
  V--> pu_AC_sec1 : Gain  Gain=1/(Sb/(Vb*sqrt(3))*sqrt(2)/2+Sb/(Vdc*2)/3)
  Out1 : Outport  VectorParamsAs1DForOutWhenUnconnected=off
  wires:
  Demux3/1 -> Sum9/1
  Demux3/2 -> Sum9/2
  Demux3/3 -> Sum10/1
  Demux3/4 -> Sum10/2
  Demux3/5 -> Sum11/1
  Sum11/1 -> Mux3/2
  Demux3/6 -> Sum11/2
  Sum9/1 -> Mux3/1
  Sum10/1 -> Mux3/3
  Mux3/1 -> Gain14/1
  V--> pu_AC_sec1/1 -> Demux3/1
  In1/1 -> V--> pu_AC_sec1/1
  Gain14/1 -> Out1/1

== system Controllers/VSC controller2/pqctrl/Ramp2 ==
  y* : Inport
  J/Psi : Gain  SaturateOnIntegerOverflow=on  OutDataTypeStr=Inherit: Same as input  ParamDataTypeStr=Inherit: Same as input
  Saturation : Saturate  UpperLimit=ramp*Ts  LowerLimit=-ramp*Ts
  Sum : Sum  Inputs=|++  InputSameDT=on  SaturateOnIntegerOverflow=on  OutDataTypeStr=Inherit: Same as first input
  Sum1 : Sum  Inputs=|+-  InputSameDT=on  SaturateOnIntegerOverflow=on  OutDataTypeStr=Inherit: Same as first input
  Unit Delay : UnitDelay  SampleTime=Ts  HasFrameUpgradeWarning=on
  yramp* : Outport  VectorParamsAs1DForOutWhenUnconnected=off
  wires:
  Unit Delay/1 -> Sum/2, Sum1/2
  y*/1 -> Sum1/1
  Sum/1 -> J/Psi/1, yramp*/1
  Saturation/1 -> Sum/1
  Sum1/1 -> Saturation/1
  J/Psi/1 -> Unit Delay/1

== system Controllers/VSC controller2/pqctrl/dq ctlr ==
  Vabcpu : Inport
  iabcpu : Inport  Port=2
  theda : Inport  Port=3
  PQrefpu : Inport  Port=4
  Demux : Demux  Outputs=2
  Gain1 : Gain  Gain=1/ks
  Mux3 : Mux  Inputs=2
  PI_d1 : powerlib_extras/Discrete  Control Blocks/Discrete PI Controller  Kp=Kp(1)  Ki=Kp(2)  Par_Limits=[1 -1]*0.15  Init=0  Ts=Ts
  PI_d2 : powerlib_extras/Discrete  Control Blocks/Discrete PI Controller  Kp=Kd(1)  Ki=Kd(2)  Par_Limits=[1 -1]*0.25  Init=0  Ts=Ts
  Subsystem1 : Subsystem
  Subtract : Sum  Inputs=+-
  Subtract1 : Sum
  Vdqref : Subsystem
  abc_dq : Subsystem
  abc_dq1 : Subsystem
  Vdqpu : Outport  VectorParamsAs1DForOutWhenUnconnected=off
  wires:
  Subsystem1/1(Idqref) -> Vdqref/2(Idqref), Subtract/1  "idqref"
  abc_dq/1(dq) -> Vdqref/1(Vdq2), Subsystem1/1(Vdq2)  "Vdq"
  abc_dq1/1(dq) -> Subtract/2  "idq"
  Subtract/1 -> Demux/1
  Demux/1 -> PI_d2/1
  Demux/2 -> PI_d1/1
  Vdqref/1(Vdqrefss) -> Subtract1/1
  PI_d2/1 -> Mux3/1
  PI_d1/1 -> Mux3/2
  Mux3/1 -> Subtract1/2
  Subtract1/1 -> Gain1/1
  Vabcpu/1 -> abc_dq/1(abc)  "vabc"
  theda/1 -> abc_dq/2(theta), abc_dq1/2(theta)
  PQrefpu/1 -> Subsystem1/2(PQref)
  iabcpu/1 -> abc_dq1/1(abc)  "iabc"
  Gain1/1 -> Vdqpu/1  "Vdqpu"

== system Controllers/VSC controller2/pqctrl/dq->abc ==
  note: Va= Vd*sinwt + Vq*cos(wt) + Vo
  note: Vb= Vd*sin(wt-2pi/3) + Vq*cos(wt-2pi/3) + Vo
  note: Vc= Vd*sin(wt+2pi/3) + Vq*cos(wt+2pi/3) + Vo
  dq : Inport
  theda : Inport  Port=2
  Fcn : Fcn  Expr=(u(1)*sin(u(3))+u(2)*cos(u(3)))
  Fcn1 : Fcn  Expr=(u(1)*sin(u(3)-2*pi/3)+u(2)*cos(u(3)-2*pi/3))
  Fcn2 : Fcn  Expr=(u(1)*sin(u(3)+2*pi/3)+u(2)*cos(u(3)+2*pi/3))
  Mux1 : Mux  Inputs=2
  Mux3 : Mux  Inputs=3
  abc : Outport  VectorParamsAs1DForOutWhenUnconnected=off
  wires:
  Fcn2/1 -> Mux3/3
  Fcn1/1 -> Mux3/2
  Fcn/1 -> Mux3/1
  Mux1/1 -> Fcn/1, Fcn2/1, Fcn1/1
  dq/1 -> Mux1/1
  theda/1 -> Mux1/2
  Mux3/1 -> abc/1  "abc"

== system Controllers/VSC controller2/pqctrl/satuation on amplitute  ==
  Vdq : Inport
  limitVdq : Inport  Port=2
  "Bias important; cancel delay in control cycle, so the PI(error) is zero, other wise PI(errer) is bais, which could over limit" : Bias  Bias=nadv*Ts*2*pi*frq  SaturateOnIntegerOverflow=off
  Complex to Magnitude-Angle : ComplexToMagnitudeAngle
  Complex to Real-Imag : ComplexToRealImag
  Demux1 : Demux  Outputs=2
  Gain : Gain  Gain=-1
  Magnitude-Angle to Complex : MagnitudeAngleToComplex
  Mux4 : Mux  Inputs=2
  Real-Imag to Complex : RealImagToComplex
  Saturation Dynamic : simulink/Discontinuities/Saturation Dynamic  OutMin=[]  OutMax=[]  OutDataTypeStr=Inherit: Same as second input  OutDataType=fixdt(1, 16)  OutScaling=2^-10  DoSatur=off
  Out1 : Outport  VectorParamsAs1DForOutWhenUnconnected=off
  wires:
  "Bias important; cancel delay in control cycle, so the PI(error) is zero, other wise PI(errer) is bais, which could over limit"/1 -> Magnitude-Angle to Complex/2
  Gain/1 -> Saturation Dynamic/3
  limitVdq/1 -> Gain/1, Saturation Dynamic/1
  Complex to Magnitude-Angle/1 -> Saturation Dynamic/2
  Saturation Dynamic/1 -> Magnitude-Angle to Complex/1
  Demux1/1 -> Real-Imag to Complex/1
  Demux1/2 -> Real-Imag to Complex/2
  Real-Imag to Complex/1 -> Complex to Magnitude-Angle/1
  Complex to Magnitude-Angle/2 -> "Bias important; cancel delay in control cycle, so the PI(error) is zero, other wise PI(errer) is bais, which could over limit"/1
  Magnitude-Angle to Complex/1 -> Complex to Real-Imag/1
  Complex to Real-Imag/2 -> Mux4/2
  Complex to Real-Imag/1 -> Mux4/1
  Mux4/1 -> Out1/1
  Vdq/1 -> Demux1/1

== system Controllers/VSC controller2/pqctrl/vipqscope ==
  note: Iacpu
  note: Iacpu
  Vac : Inport
  Iac : Inport  Port=2
  pqref : Inport  Port=3
  3-phase Instantaneous Active & Reactive Power : powerlib_extras/Measurements/3-phase  Instantaneous  Active & Reactive Power
  Demux1 : Demux  Outputs=2
  Demux2 : Demux  Outputs=2
  Gain2 : Gain  Gain=2/3
  Mux1 : Mux  Inputs=2
  Mux3 : Mux  Inputs=2
  vipq : Scope  Commented=on  NumInputPorts=4
  wires:
  Mux1/1 -> vipq/3  "p"
  Mux3/1 -> vipq/4  "q"
  Demux2/2 -> Mux3/2
  Demux2/1 -> Mux1/2
  Gain2/1 -> Demux2/1
  3-phase Instantaneous Active & Reactive Power/1 -> Gain2/1
  Demux1/1 -> Mux1/1
  Vac/1 -> vipq/1, 3-phase Instantaneous Active & Reactive Power/1  "Vacpu"
  Iac/1 -> vipq/2, 3-phase Instantaneous Active & Reactive Power/2
  Demux1/2 -> Mux3/1
  pqref/1 -> Demux1/1

== system Controllers/pulsegen_VBC1/VBC/VBC1 ==
  mode : Inport
  g : Inport  Port=2
  Vc : Inport  Port=3
  ichg : Inport  Port=4
  Nref : Inport  Port=5
  Constant : Constant  Value=numberOfCell
  Demux3 : Demux  Outputs=2
  MATLAB Function : MATLAB Function  TreatAsAtomicUnit=on
  Signal Specification : SignalSpecification  Dimensions=2
  Terminator : Terminator
  Unit Delay : UnitDelay  SampleTime=Ts  HasFrameUpgradeWarning=on
  Unit Delay1 : UnitDelay  SampleTime=Ts  HasFrameUpgradeWarning=on
  go : Outport  VectorParamsAs1DForOutWhenUnconnected=off
  wires:
  Signal Specification/1 -> Unit Delay/1
  g/1 -> MATLAB Function/1(gate_in)
  Vc/1 -> MATLAB Function/2(Vc)
  ichg/1 -> MATLAB Function/3(ichg)
  MATLAB Function/1(go) -> go/1, Unit Delay1/1
  MATLAB Function/2(int) -> Signal Specification/1
  Nref/1 -> MATLAB Function/4(Nref)
  mode/1 -> Demux3/1
  Demux3/2 -> MATLAB Function/5(errV)
  Unit Delay/1 -> MATLAB Function/7(inti)
  Unit Delay1/1 -> MATLAB Function/6(g_his)
  Demux3/1 -> Terminator/1
  Constant/1 -> MATLAB Function/8(nbc)

== system Controllers/pulsegen_VBC1/VBC/VBC2 ==
  mode : Inport
  g : Inport  Port=2
  Vc : Inport  Port=3
  ichg : Inport  Port=4
  Nref : Inport  Port=5
  Constant : Constant  Value=numberOfCell
  Demux3 : Demux  Outputs=2
  MATLAB Function : MATLAB Function  TreatAsAtomicUnit=on
  Signal Specification : SignalSpecification  Dimensions=2
  Terminator : Terminator
  Unit Delay : UnitDelay  SampleTime=Ts  HasFrameUpgradeWarning=on
  Unit Delay1 : UnitDelay  SampleTime=Ts  HasFrameUpgradeWarning=on
  go : Outport  VectorParamsAs1DForOutWhenUnconnected=off
  wires:
  Constant/1 -> MATLAB Function/8(nbc)
  Demux3/1 -> Terminator/1
  Unit Delay1/1 -> MATLAB Function/6(g_his)
  Unit Delay/1 -> MATLAB Function/7(inti)
  Demux3/2 -> MATLAB Function/5(errV)
  mode/1 -> Demux3/1
  Nref/1 -> MATLAB Function/4(Nref)
  MATLAB Function/2(int) -> Signal Specification/1
  MATLAB Function/1(go) -> Unit Delay1/1, go/1
  ichg/1 -> MATLAB Function/3(ichg)
  Vc/1 -> MATLAB Function/2(Vc)
  g/1 -> MATLAB Function/1(gate_in)
  Signal Specification/1 -> Unit Delay/1

== system Controllers/pulsegen_VBC1/VBC/VBC3 ==
  mode : Inport
  g : Inport  Port=2
  Vc : Inport  Port=3
  ichg : Inport  Port=4
  Nref : Inport  Port=5
  Constant : Constant  Value=numberOfCell
  Demux3 : Demux  Outputs=2
  MATLAB Function : MATLAB Function  TreatAsAtomicUnit=on
  Signal Specification : SignalSpecification  Dimensions=2
  Terminator : Terminator
  Unit Delay : UnitDelay  SampleTime=Ts  HasFrameUpgradeWarning=on
  Unit Delay1 : UnitDelay  SampleTime=Ts  HasFrameUpgradeWarning=on
  go : Outport  VectorParamsAs1DForOutWhenUnconnected=off
  wires:
  Constant/1 -> MATLAB Function/8(nbc)
  Demux3/1 -> Terminator/1
  Unit Delay1/1 -> MATLAB Function/6(g_his)
  Unit Delay/1 -> MATLAB Function/7(inti)
  Demux3/2 -> MATLAB Function/5(errV)
  mode/1 -> Demux3/1
  Nref/1 -> MATLAB Function/4(Nref)
  MATLAB Function/2(int) -> Signal Specification/1
  MATLAB Function/1(go) -> Unit Delay1/1, go/1
  ichg/1 -> MATLAB Function/3(ichg)
  Vc/1 -> MATLAB Function/2(Vc)
  g/1 -> MATLAB Function/1(gate_in)
  Signal Specification/1 -> Unit Delay/1

== system Controllers/pulsegen_VBC1/VBC/VBC4 ==
  mode : Inport
  g : Inport  Port=2
  Vc : Inport  Port=3
  ichg : Inport  Port=4
  Nref : Inport  Port=5
  Constant : Constant  Value=numberOfCell
  Demux3 : Demux  Outputs=2
  MATLAB Function : MATLAB Function  TreatAsAtomicUnit=on
  Signal Specification : SignalSpecification  Dimensions=2
  Terminator : Terminator
  Unit Delay : UnitDelay  SampleTime=Ts  HasFrameUpgradeWarning=on
  Unit Delay1 : UnitDelay  SampleTime=Ts  HasFrameUpgradeWarning=on
  go : Outport  VectorParamsAs1DForOutWhenUnconnected=off
  wires:
  Signal Specification/1 -> Unit Delay/1
  g/1 -> MATLAB Function/1(gate_in)
  Vc/1 -> MATLAB Function/2(Vc)
  ichg/1 -> MATLAB Function/3(ichg)
  MATLAB Function/1(go) -> go/1, Unit Delay1/1
  MATLAB Function/2(int) -> Signal Specification/1
  Nref/1 -> MATLAB Function/4(Nref)
  mode/1 -> Demux3/1
  Demux3/2 -> MATLAB Function/5(errV)
  Unit Delay/1 -> MATLAB Function/7(inti)
  Unit Delay1/1 -> MATLAB Function/6(g_his)
  Demux3/1 -> Terminator/1
  Constant/1 -> MATLAB Function/8(nbc)

== system Controllers/pulsegen_VBC1/VBC/VBC5 ==
  mode : Inport
  g : Inport  Port=2
  Vc : Inport  Port=3
  ichg : Inport  Port=4
  Nref : Inport  Port=5
  Constant : Constant  Value=numberOfCell
  Demux3 : Demux  Outputs=2
  MATLAB Function : MATLAB Function  TreatAsAtomicUnit=on
  Signal Specification : SignalSpecification  Dimensions=2
  Terminator : Terminator
  Unit Delay : UnitDelay  SampleTime=Ts  HasFrameUpgradeWarning=on
  Unit Delay1 : UnitDelay  SampleTime=Ts  HasFrameUpgradeWarning=on
  go : Outport  VectorParamsAs1DForOutWhenUnconnected=off
  wires:
  Constant/1 -> MATLAB Function/8(nbc)
  Demux3/1 -> Terminator/1
  Unit Delay1/1 -> MATLAB Function/6(g_his)
  Unit Delay/1 -> MATLAB Function/7(inti)
  Demux3/2 -> MATLAB Function/5(errV)
  mode/1 -> Demux3/1
  Nref/1 -> MATLAB Function/4(Nref)
  MATLAB Function/2(int) -> Signal Specification/1
  MATLAB Function/1(go) -> Unit Delay1/1, go/1
  ichg/1 -> MATLAB Function/3(ichg)
  Vc/1 -> MATLAB Function/2(Vc)
  g/1 -> MATLAB Function/1(gate_in)
  Signal Specification/1 -> Unit Delay/1

== system Controllers/pulsegen_VBC1/VBC/VBC6 ==
  mode : Inport
  g : Inport  Port=2
  Vc : Inport  Port=3
  ichg : Inport  Port=4
  Nref : Inport  Port=5
  Constant : Constant  Value=numberOfCell
  Demux3 : Demux  Outputs=2
  MATLAB Function : MATLAB Function  TreatAsAtomicUnit=on
  Signal Specification : SignalSpecification  Dimensions=2
  Terminator : Terminator
  Unit Delay : UnitDelay  SampleTime=Ts  HasFrameUpgradeWarning=on
  Unit Delay1 : UnitDelay  SampleTime=Ts  HasFrameUpgradeWarning=on
  go : Outport  VectorParamsAs1DForOutWhenUnconnected=off
  wires:
  Signal Specification/1 -> Unit Delay/1
  g/1 -> MATLAB Function/1(gate_in)
  Vc/1 -> MATLAB Function/2(Vc)
  ichg/1 -> MATLAB Function/3(ichg)
  MATLAB Function/1(go) -> go/1, Unit Delay1/1
  MATLAB Function/2(int) -> Signal Specification/1
  Nref/1 -> MATLAB Function/4(Nref)
  mode/1 -> Demux3/1
  Demux3/2 -> MATLAB Function/5(errV)
  Unit Delay/1 -> MATLAB Function/7(inti)
  Unit Delay1/1 -> MATLAB Function/6(g_his)
  Demux3/1 -> Terminator/1
  Constant/1 -> MATLAB Function/8(nbc)

== system Controllers/pulsegen_VBC1/pulse_gen/Carrier_generatorgood ==
  Constant : Constant  Value=[1:nb_mod]/(fc*nb_mod)
  Constant1 : Constant  Value=ceil([[1:nb_mod]/(fc*nb_mod)]/Ts)
  Display1 : Display
  Repeating Sequence2 : simulink/Sources/Repeating Sequence  rep_seq_t=[0 1/2 1]/fx  rep_seq_y=[1 -1 1]
  Selector : Selector  Commented=on  InputPortWidth=1  IndexOptions=Index vector (dialog)  Indices=[ones(100,1)]  OutputSizes=1
  Variable Transport Delay1 : VariableTransportDelay  Commented=on  MaximumPoints=9216  FixedBuffer=on  ZeroDelay=on  TransDelayFeedthrough=on
  Variable Transport Delay2 : VariableTransportDelay  MaximumPoints=9216  FixedBuffer=on  ZeroDelay=on  TransDelayFeedthrough=on
  Out1 : Outport  VectorParamsAs1DForOutWhenUnconnected=off
  wires:
  Constant1/1 -> Display1/1
  Variable Transport Delay2/1 -> Out1/1
  Repeating Sequence2/1 -> Variable Transport Delay2/1
  Constant/1 -> Variable Transport Delay2/2

== system Controllers/pulsegen_VBC1/pulse_gen/PWM ==
  carrier : Inport
  Vcell_ref : Inport  Port=2
  pgmode : Inport  Port=3
  Data Type Conversion : DataTypeConversion  OutDataTypeStr=double  SaturateOnIntegerOverflow=off  RndMeth=Floor
  NLC : Subsystem
  Relational Operator : RelationalOperator  Operator=>  OutDataTypeStr=boolean  RndMeth=Simplest  InputSameDT=off
  Terminator : Terminator
  phase_reorder6 : Selector  InputPortWidth=6  IndexOptions=Index vector (dialog)  Indices=reshape(ones(numberOfCell,1)*[1:6],1,[])  OutputSizes=1
  Upper_gate : Outport  VectorParamsAs1DForOutWhenUnconnected=off
  NLCref : Outport  Port=2  VectorParamsAs1DForOutWhenUnconnected=off
  wires:
  pgmode/1 -> Terminator/1
  Data Type Conversion/1 -> Upper_gate/1
  Relational Operator/1 -> Data Type Conversion/1
  phase_reorder6/1 -> Relational Operator/1
  carrier/1 -> Relational Operator/2
  Vcell_ref/1 -> phase_reorder6/1, NLC/1(In1)
  NLC/1(Out1) -> NLCref/1

== system Controllers/pulsegen_VBC1/pulse_gen/carrier_gen ==
  Constant : Constant  DisableCoverage=on  Value=period
  Digital Clock : DigitalClock  SampleTime=Ts
  Look-Up Table1 : Lookup_n-D  DisableCoverage=on  NumberOfTableDimensions=1  BreakpointsForDimension1=rep_seq_t - min(rep_seq_t)  BreakpointsForDimension3=[5, 7]  Table=rep_seq_y  InternalRulePriority=Speed  SaturateOnIntegerOverflow=on
  Math Function : Math  DisableCoverage=on  Operator=mod  SignedPower=on
  Output : SignalConversion  OverrideOpt=off
  Sum : Sum  DisableCoverage=on  Inputs=+-+  InputSameDT=on  SaturateOnIntegerOverflow=on  OutDataTypeStr=Inherit: Same as first input
  offset : Constant  DisableCoverage=on  Value=Noffset
  startTime : S-Function  Commented=on  DisableCoverage=on  FunctionName=sfun_tstart  SFunctionDeploymentMode=off  EnableBusSupport=off
  Out1 : Outport  VectorParamsAs1DForOutWhenUnconnected=off
  wires:
  Sum/1 -> Math Function/1
  Output/1 -> Out1/1
  offset/1 -> Sum/3
  Math Function/1 -> Look-Up Table1/1
  Digital Clock/1 -> Sum/1
  startTime/1 -> Sum/2
  Look-Up Table1/1 -> Output/1
  Constant/1 -> Math Function/2

== system Controllers/pulsegen_VBC2/VBC/VBC1 ==
  mode : Inport
  g : Inport  Port=2
  Vc : Inport  Port=3
  ichg : Inport  Port=4
  Nref : Inport  Port=5
  Constant : Constant  Value=numberOfCell
  Demux3 : Demux  Outputs=2
  MATLAB Function : MATLAB Function  TreatAsAtomicUnit=on
  Signal Specification : SignalSpecification  Dimensions=2
  Terminator : Terminator
  Unit Delay : UnitDelay  SampleTime=Ts  HasFrameUpgradeWarning=on
  Unit Delay1 : UnitDelay  SampleTime=Ts  HasFrameUpgradeWarning=on
  go : Outport  VectorParamsAs1DForOutWhenUnconnected=off
  wires:
  Constant/1 -> MATLAB Function/8(nbc)
  Demux3/1 -> Terminator/1
  Unit Delay1/1 -> MATLAB Function/6(g_his)
  Unit Delay/1 -> MATLAB Function/7(inti)
  Demux3/2 -> MATLAB Function/5(errV)
  mode/1 -> Demux3/1
  Nref/1 -> MATLAB Function/4(Nref)
  MATLAB Function/2(int) -> Signal Specification/1
  MATLAB Function/1(go) -> Unit Delay1/1, go/1
  ichg/1 -> MATLAB Function/3(ichg)
  Vc/1 -> MATLAB Function/2(Vc)
  g/1 -> MATLAB Function/1(gate_in)
  Signal Specification/1 -> Unit Delay/1

== system Controllers/pulsegen_VBC2/VBC/VBC2 ==
  mode : Inport
  g : Inport  Port=2
  Vc : Inport  Port=3
  ichg : Inport  Port=4
  Nref : Inport  Port=5
  Constant : Constant  Value=numberOfCell
  Demux3 : Demux  Outputs=2
  MATLAB Function : MATLAB Function  TreatAsAtomicUnit=on
  Signal Specification : SignalSpecification  Dimensions=2
  Terminator : Terminator
  Unit Delay : UnitDelay  SampleTime=Ts  HasFrameUpgradeWarning=on
  Unit Delay1 : UnitDelay  SampleTime=Ts  HasFrameUpgradeWarning=on
  go : Outport  VectorParamsAs1DForOutWhenUnconnected=off
  wires:
  Signal Specification/1 -> Unit Delay/1
  g/1 -> MATLAB Function/1(gate_in)
  Vc/1 -> MATLAB Function/2(Vc)
  ichg/1 -> MATLAB Function/3(ichg)
  MATLAB Function/1(go) -> go/1, Unit Delay1/1
  MATLAB Function/2(int) -> Signal Specification/1
  Nref/1 -> MATLAB Function/4(Nref)
  mode/1 -> Demux3/1
  Demux3/2 -> MATLAB Function/5(errV)
  Unit Delay/1 -> MATLAB Function/7(inti)
  Unit Delay1/1 -> MATLAB Function/6(g_his)
  Demux3/1 -> Terminator/1
  Constant/1 -> MATLAB Function/8(nbc)

== system Controllers/pulsegen_VBC2/VBC/VBC3 ==
  mode : Inport
  g : Inport  Port=2
  Vc : Inport  Port=3
  ichg : Inport  Port=4
  Nref : Inport  Port=5
  Constant : Constant  Value=numberOfCell
  Demux3 : Demux  Outputs=2
  MATLAB Function : MATLAB Function  TreatAsAtomicUnit=on
  Signal Specification : SignalSpecification  Dimensions=2
  Terminator : Terminator
  Unit Delay : UnitDelay  SampleTime=Ts  HasFrameUpgradeWarning=on
  Unit Delay1 : UnitDelay  SampleTime=Ts  HasFrameUpgradeWarning=on
  go : Outport  VectorParamsAs1DForOutWhenUnconnected=off
  wires:
  Constant/1 -> MATLAB Function/8(nbc)
  Demux3/1 -> Terminator/1
  Unit Delay1/1 -> MATLAB Function/6(g_his)
  Unit Delay/1 -> MATLAB Function/7(inti)
  Demux3/2 -> MATLAB Function/5(errV)
  mode/1 -> Demux3/1
  Nref/1 -> MATLAB Function/4(Nref)
  MATLAB Function/2(int) -> Signal Specification/1
  MATLAB Function/1(go) -> Unit Delay1/1, go/1
  ichg/1 -> MATLAB Function/3(ichg)
  Vc/1 -> MATLAB Function/2(Vc)
  g/1 -> MATLAB Function/1(gate_in)
  Signal Specification/1 -> Unit Delay/1
